simulink model "test03"  (R2025b)
settings: Solver=VariableStepAuto  StartTime=0.0  StopTime=60  RelTol=1e-3
settings Model: Creator=sanborkl  LastModifiedBy=sanborkl

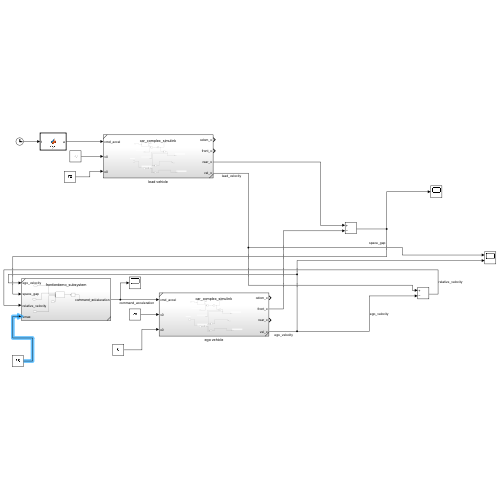
[thumbnail: Simulink's stored preview of the top-level diagram]
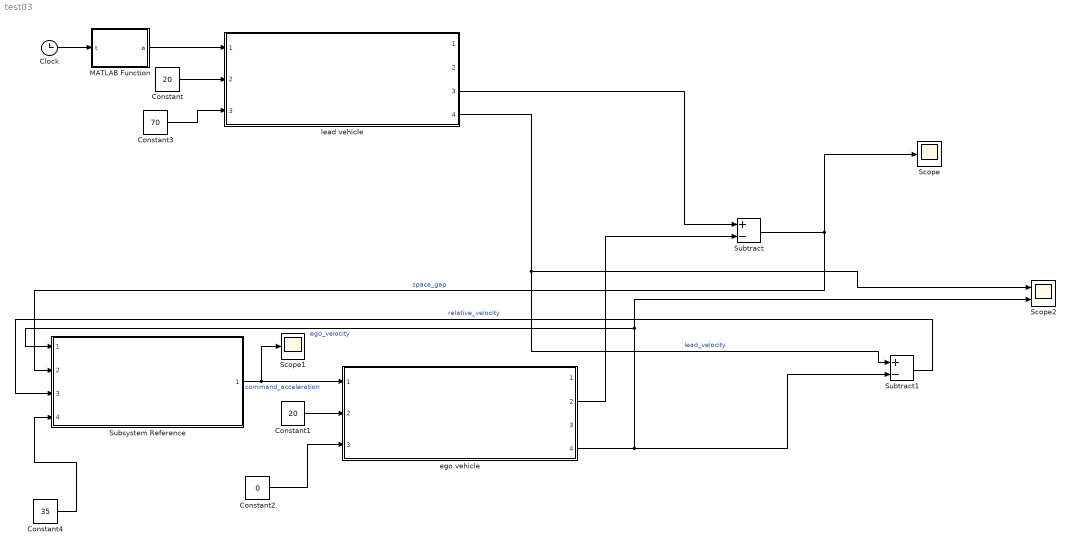
== system test03 ==
  Clock : Clock
  Constant : Constant  Value=20
  Constant1 : Constant  Value=20
  Constant2 : Constant  Value=0
  Constant3 : Constant  Value=70
  Constant4 : Constant  Value=35
  MATLAB Function : MATLAB Function  TreatAsAtomicUnit=on
  Scope : Scope
      settings: ActiveDisplayYMinimum=0.38343831402384776  ActiveDisplayYMaximum=51.068506853997349
  Scope1 : Scope
      settings: ActiveDisplayYMinimum=-0.48058103190538431  ActiveDisplayYMaximum=0.58595776634763919
  Scope2 : Scope  NumInputPorts=2
      settings: ActiveDisplayYMinimum=15.35010288755884  ActiveDisplayYMaximum=22.397939343925227  DataLoggingVariableName=ScopeData2
  Subsystem Reference : Subsystem  ReferencedSubsystem=frontierdemo_subsystem
  Subtract : Sum  Inputs=+-
  Subtract1 : Sum  Inputs=+-
  ego vehicle : Subsystem  ReferencedSubsystem=car_complex_simulink
  lead vehicle : Subsystem  ReferencedSubsystem=car_complex_simulink
  wires:
  Constant2/1 -> ego vehicle/3
  Constant3/1 -> lead vehicle/3
  ego vehicle/2 -> Subtract/2
  MATLAB Function/1(a) -> lead vehicle/1
  ego vehicle/4 -> Scope2/2, Subsystem Reference/1, Subtract1/2  "ego_velocity"
  lead vehicle/4 -> Scope2/1, Subtract1/1  "lead_velocity"
  lead vehicle/3 -> Subtract/1
  Constant1/1 -> ego vehicle/2
  Subtract1/1 -> Subsystem Reference/3  "relative_velocity"
  Constant/1 -> lead vehicle/2
  Subsystem Reference/1 -> Scope1/1, ego vehicle/1  "command_acceleration"
  Subtract/1 -> Subsystem Reference/2, Scope/1  "space_gap"
  Clock/1 -> MATLAB Function/1(t)
  Constant4/1 -> Subsystem Reference/4

== matlab function test03/MATLAB Function ==
  data: t input; a output
function a = fcn(t)

a = sin(t);
